simulink model "model_main_duty"  (R2024b)
settings: Solver=ode4  StartTime=0.0  StopTime=1000  FixedStep=dt  RelTol=1e-3
InitFcn:
  | model_init
undefined symbols (not defined in the file): dt, Iws, m_tot, norm_Ib, Omega1_init, Omega2_init, Omega3_init, Omega4_init, Omega_ref, qb0, rad2rpm, RCS_F, RCS_F_vec, RCS_Pos, RCS_pos, RCS_PWM_Freq, RCS_Sampling_time, RCS_THR_vec, REL_TS_POS_I_0, REL_TS_VEL_I_0, RW_As, RW_Max_Speed, RW_t_max, SC_Ib, SC_state0, SS_Total_Mass, TC_Kepler, TS_Ib, TS_qb0, TS_state0, TS_wb0, wb0
libraries: simulink_extras x17, simulink x16, sharedtransform x11, aerolibutil x10
(part 1 of 3)
settings Model: PacingRate=1.100000  Creator=yhj2019  LastModifiedBy=ASCL
settings DebuggingCC: UnderSpecifiedDimensionMsg=warning
settings RTWCC: GPUComputeCapability=3.5

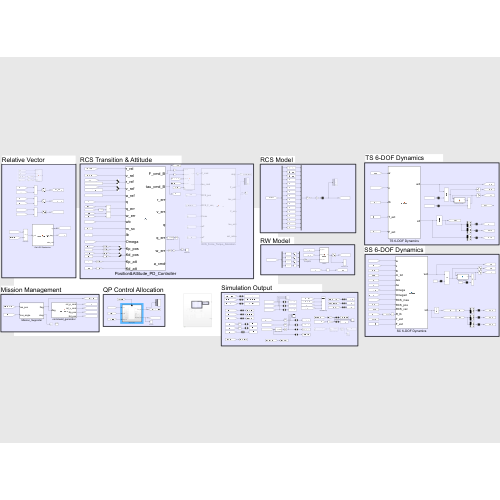
[thumbnail: Simulink's stored preview of the top-level diagram]
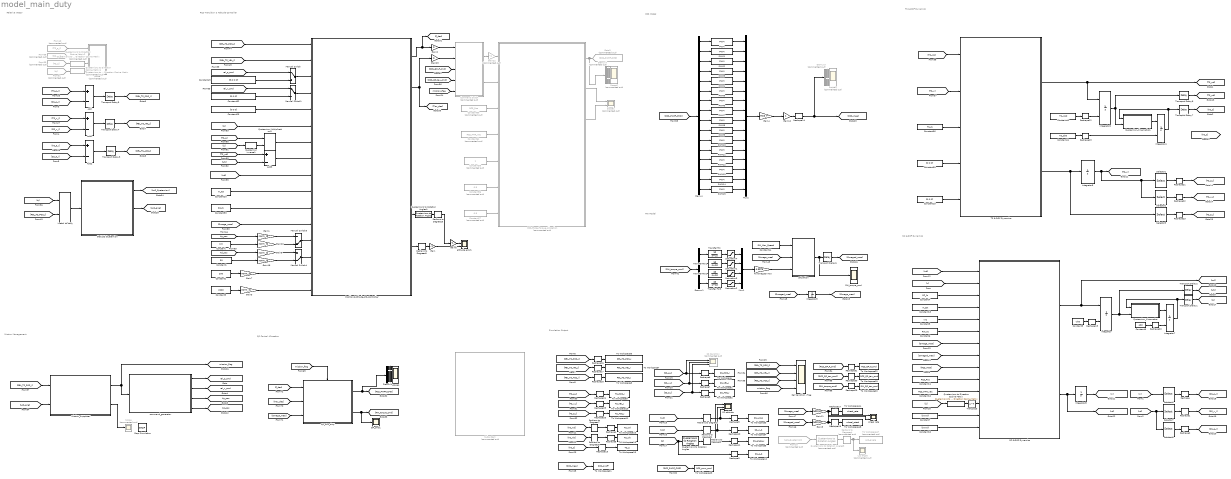
== system model_main_duty ==
  note: TS 6-DOF Dynamics
  note: RW Model
  note: RCS Model
  note: Simulation Output
  note: RCS Transition & Attitude Controller
  note: SS 6-DOF Dynamics
  note: Relative Vector
  note: Mission Management
  note: QP Control Allocation
  Add{,1..3} (4 alike) : Sum  Inputs=+-
  Command Switch : MATLAB Function  Commented=on  TreatAsAtomicUnit=on
  Constant : Constant  Value=0.3
  Constant1 : Constant  Value=30
  Constant{7,10,15,23,39,52} (6 alike) : Constant  Value=[0 0 0]'
  Constant11 : Constant  Value=RCS_Pos
  Constant12 : Constant  Value=RCS_THR_vec
  Constant13 : Constant  Value=m_tot
  Constant14 : Constant  Value=RW_Max_Speed
  Constant2 : Constant  Value=200
  Constant20 : Constant  Value=m_tot
  Constant3 : Constant  Value=2000
  Constant36 : Constant  Value=TS_Ib
  Constant4 : Constant  Value=SC_Ib
  Constant40 : Constant  Value=TS_wb0
  Constant41 : Constant  Value=TS_qb0
  Constant49 : Constant  Value=[5.0 0 0]'
  Constant5 : Constant  Value=Iws
  Constant53 : Constant  Value=SC_Ib
  Constant55 : Constant  Commented=on
  Constant56 : Constant  Commented=on  Value=0.5
  Constant57 : Constant  Commented=on  Value=0.5
  Constant6 : Constant  Value=RW_As
  Constant60 : Constant  Commented=on  Value=RCS_Pos
  Constant61 : Constant  Commented=on  Value=RCS_THR_vec
  Constant8 : Constant  Value=wb0
  Constant9 : Constant  Value=qb0
  Demux : Demux  Outputs=16
  Demux1 : Demux
  Demux2 : Demux  Commented=on  Outputs=16
  Demux3 : Demux  Commented=on  Outputs=16
  Demux4 : Demux  Outputs=16
  From10 : From  Commented=on  GotoTag=LoS_Quaternion
  From31 : From  Commented=on  GotoTag=q
  From39 : From  Commented=on  GotoTag=TS_q
  From40 : From  Commented=on  GotoTag=TS_p_I
  From68 : From  Commented=on  GotoTag=SS_p_I
  Gain : Gain  Gain=-1
  Gain{1,3,5,7,18,20} (6 alike) : Gain  Gain=norm_Ib
  Gain11 : Gain  Gain=rad2rpm
  Gain12 : Gain
  Gain2 : Gain  Gain=0
  Gain22 : Gain  Commented=on  Gain=-1
  Gain23 : Gain  Gain=0
  Gain4 : Gain  Gain=RCS_F
  Gain6 : Gain  Gain=-1
  Gain8 : Gain  Gain=rad2rpm
  Get LOS Quaternion : MATLAB Function  TreatAsAtomicUnit=on
  Goto3 : Goto  Commented=on  GotoTag=RCS_PWPF_CMD
  Inetial to body : aerolibutil/Quaternion Rotation
  Integrator : Integrator  InitialConditionSource=external  InitialCondition=wb0
  Integrator2 : Integrator  InitialConditionSource=external  InitialCondition=wb0
  Integrator3 : Integrator  InitialCondition=[Omega1_init Omega2_init Omega3_init Omega4_init]'
  Integrator4 : Integrator  InitialConditionSource=external
  Integrator5 : Integrator  InitialCondition=TS_state0'
  Integrator7 : Integrator  InitialConditionSource=external
  Integrator8 : Integrator  InitialCondition=SC_state0'
  Los angle : Scope  Commented=on
  Manual Switch : ManualSwitch
  Manual Switch1 : ManualSwitch
  Manual Switch3 : ManualSwitch  CurrentSetting=0
  Manual Switch4 : ManualSwitch  CurrentSetting=0
  Mission_Supporter : MATLAB Function  TreatAsAtomicUnit=on
  Mux1 : Mux
  Mux2 : Mux  Inputs=16
  PWM{,1..15} (16 alike) : simulink/Discontinuities/PWM  DisableCoverage=on  Period=RCS_PWM_Freq  InitialDelay=0  DisallowZeroDutyCycle=off  RunAtFixedTimeIntervals=on  SampleTime=RCS_Sampling_time
  Position&Attitude_PD_Controller : MATLAB Function  TreatAsAtomicUnit=on
  QP_RCS_duty : Subsystem  TreatAsAtomicUnit=on
  QP_cmd1 : Scope
  Quaternion Inverse1 : aerolibutil/Quaternion Inverse
  Quaternion Multiplication3 : aerolibutil/Quaternion Multiplication
  Quaternion_Kinematics : MATLAB Function  TreatAsAtomicUnit=on
  Quaternion_Kinematics1 : MATLAB Function  TreatAsAtomicUnit=on
  Quaternions to Direction Cosine Matrix : sharedtransform/Quaternions to  Direction Cosine Matrix  aMode=aMode
      settings: LibrarySourceBlock=|
      | aerolibtransform2/Quaternions to
      | Direction Cosine Matrix
  Quaternions to Direction Cosine Matrix1 : sharedtransform/Quaternions to  Direction Cosine Matrix  Commented=on  aMode=aMode
      settings: LibrarySourceBlock=|
      | aerolibtransform2/Quaternions to
      | Direction Cosine Matrix
  Quaternions to Direction Cosine Matrix2 : sharedtransform/Quaternions to  Direction Cosine Matrix  Commented=on  aMode=aMode
      settings: LibrarySourceBlock=|
      | aerolibtransform2/Quaternions to
      | Direction Cosine Matrix
  Quaternions to Rotation Angles : sharedtransform/Quaternions to Rotation Angles  rotationOrder=ZYX  aMode=aMode
  Quaternions to Rotation Angles1 : sharedtransform/Quaternions to Rotation Angles  rotationOrder=ZYX  aMode=aMode
  Quaternions to Rotation Angles3 : sharedtransform/Quaternions to Rotation Angles  Commented=on  rotationOrder=ZYX  aMode=aMode
  RCS_Force_Torque_Allocation : MATLAB Function  Commented=on  TreatAsAtomicUnit=on
  RW_torque_cmd : Scope
  Radians to Degrees{,1..3,7..9} (7 alike) : simulink_extras/Transformations/Radians to Degrees
  Radians to Degrees4 : simulink_extras/Transformations/Radians to Degrees  Commented=on
  Rel transition / flag : Scope  NumInputPorts=4
  Reshape{,1..2,12..14,19..23} (11 alike) : Reshape  OutputDimensionality=Column vector (2-D)
  Reshape{3..11,15..18,24..31} (21 alike) : Reshape  OutputDimensionality=Row vector (2-D)
  SC 6-DOF Dynamics : MATLAB Function  TreatAsAtomicUnit=on
  SS attitude : Scope  NumInputPorts=3
  SS transition : Scope  Commented=on  NumInputPorts=3
  Saturation{1..4} (4 alike) : Saturate  UpperLimit=RW_t_max  LowerLimit=-RW_t_max
  Scope : Scope  Commented=on
  Scope1 : Scope  Commented=on  NumInputPorts=2
  Scope2 : Scope  Commented=on  NumInputPorts=16
  Scope3 : Scope  Commented=on  NumInputPorts=16
  Scope4 : Scope  NumInputPorts=16
  Selector1 : Selector  InputPortWidth=6  IndexOptions=Index vector (dialog)  Indices=[1 2 3]  OutputSizes=1
  Selector2 : Selector  InputPortWidth=6  IndexOptions=Index vector (dialog)  Indices=[4 5 6]  OutputSizes=1
  Selector6 : Selector  InputPortWidth=6  IndexOptions=Index vector (dialog)  Indices=[1 2 3]  OutputSizes=1
  Selector7 : Selector  InputPortWidth=6  IndexOptions=Index vector (dialog)  Indices=[1 2 3]  OutputSizes=1
  Selector8 : Selector  InputPortWidth=6  IndexOptions=Index vector (dialog)  Indices=[4 5 6]  OutputSizes=1
  Selector9 : Selector  InputPortWidth=6  IndexOptions=Index vector (dialog)  Indices=[4 5 6]  OutputSizes=1
  Stop Simulation : Stop
  Subsystem : Subsystem  Commented=on
  TS 6-DOF Dynamics : MATLAB Function  TreatAsAtomicUnit=on
  To OmegaD max : Gain  Gain=4.3975
  To Workspace : ToWorkspace  VariableName=SS_POS_I  SampleTime=-1
      settings: Save2DSignal=2-D array (concatenate along first dimension)
  To Workspace1 : ToWorkspace  VariableName=SS_VEL_I  SampleTime=-1
      settings: Save2DSignal=2-D array (concatenate along first dimension)
  To Workspace10 : ToWorkspace  VariableName=TS_VEL_I  SampleTime=-1
      settings: Save2DSignal=2-D array (concatenate along first dimension)
  To Workspace11 : ToWorkspace  VariableName=TS_ACC_I  SampleTime=-1
      settings: Save2DSignal=2-D array (concatenate along first dimension)
  To Workspace12 : ToWorkspace  VariableName=SS_q_b  SampleTime=-1
      settings: Save2DSignal=2-D array (concatenate along first dimension)
  To Workspace13 : ToWorkspace  VariableName=TS_wb  SampleTime=-1
      settings: Save2DSignal=2-D array (concatenate along first dimension)
  To Workspace14 : ToWorkspace  VariableName=wheel_rate  SampleTime=-1
      settings: Save2DSignal=2-D array (concatenate along first dimension)
  To Workspace15 : ToWorkspace  VariableName=TS_q  SampleTime=-1
      settings: Save2DSignal=2-D array (concatenate along first dimension)
  To Workspace16 : ToWorkspace  VariableName=TS_wd  SampleTime=-1
      settings: Save2DSignal=2-D array (concatenate along first dimension)
  To Workspace17 : ToWorkspace  Commented=on  VariableName=LoS_angle  SampleTime=-1
      settings: Save2DSignal=2-D array (concatenate along first dimension)
  To Workspace18 : ToWorkspace  VariableName=wheel_rated  SampleTime=-1
      settings: Save2DSignal=2-D array (concatenate along first dimension)
  To Workspace19 : ToWorkspace  VariableName=RCS_QP_tau_cmd  SampleTime=-1
      settings: Save2DSignal=2-D array (concatenate along first dimension)
  To Workspace2 : ToWorkspace  VariableName=SS_ACC_I  SampleTime=-1
      settings: Save2DSignal=2-D array (concatenate along first dimension)
  To Workspace20 : ToWorkspace  VariableName=RW_QP_tau_cmd  SampleTime=-1
      settings: Save2DSignal=2-D array (concatenate along first dimension)
  To Workspace21 : ToWorkspace  VariableName=RCS_onoff  SaveFormat=Timeseries  SampleTime=-1
  To Workspace22 : ToWorkspace  VariableName=RCS_QP_F_cmd  SampleTime=-1
      settings: Save2DSignal=2-D array (concatenate along first dimension)
  To Workspace23 : ToWorkspace  VariableName=RCS_pwm_cmd  SaveFormat=Timeseries  SampleTime=-1
  To Workspace3 : ToWorkspace  VariableName=SS_wd_b  SampleTime=-1
      settings: Save2DSignal=2-D array (concatenate along first dimension)
  To Workspace4 : ToWorkspace  VariableName=SS_w_b  SampleTime=-1
      settings: Save2DSignal=2-D array (concatenate along first dimension)
  To Workspace5 : ToWorkspace  VariableName=SS_angle_I  SampleTime=-1
      settings: Save2DSignal=2-D array (concatenate along first dimension)
  To Workspace6 : ToWorkspace  VariableName=REL_TS_POS_I  SampleTime=-1
      settings: Save2DSignal=2-D array (concatenate along first dimension)
  To Workspace7 : ToWorkspace  VariableName=REL_TS_VEL_I  SampleTime=-1
      settings: Save2DSignal=2-D array (concatenate along first dimension)
  To Workspace8 : ToWorkspace  VariableName=REL_TS_ACC_I  SampleTime=-1
      settings: Save2DSignal=2-D array (concatenate along first dimension)
  To Workspace9 : ToWorkspace  VariableName=TS_POS_I  SampleTime=-1
      settings: Save2DSignal=2-D array (concatenate along first dimension)
  Transfer Fcn{,1..3} (4 alike) : TransferFcn  Numerator=[10]  Denominator=[1 10]
  Transport Delay1 : TransportDelay  DelayTime=dt  InitialOutput=qb0
  Transport Delay2 : TransportDelay  DelayTime=dt  InitialOutput=wb0
  Transport Delay3 : TransportDelay  DelayTime=dt  InitialOutput=[0 0 0]'
  Transport Delay4 : TransportDelay  DelayTime=dt  InitialOutput=REL_TS_VEL_I_0
  Transport Delay5 : TransportDelay  DelayTime=dt  InitialOutput=REL_TS_POS_I_0
  Transport Delay6 : TransportDelay  DelayTime=dt  InitialOutput=[0 0 0 0]'
  Transport Delay7 : TransportDelay  DelayTime=dt  InitialOutput=TS_qb0
  Transport Delay8 : TransportDelay  DelayTime=dt  InitialOutput=TS_wb0
  Transpose : Math  Operator=transpose
  attitude error1 : Scope  NumInputPorts=2
  command_generator : MATLAB Function  TreatAsAtomicUnit=on
  probe : MATLAB Function  Commented=on  TreatAsAtomicUnit=on
  saturation : MATLAB Function  TreatAsAtomicUnit=on
  wheel rate : Scope  NumInputPorts=2
  tag scope: Kd_pos=global, Kp_pos=global, mission_flag=global, rel_p_cmd=global, rel_v_cmd=global
  wires:
  Reshape6/1 -> To Workspace/1
  Reshape7/1 -> To Workspace1/1
  Reshape8/1 -> To Workspace2/1
  [TS_p_I] -> Add/1
  [SS_p_I] -> Add/2
  [SS_v_I] -> Add1/2
  [TS_v_I] -> Add1/1
  [SS_a_I] -> Add2/2
  [TS_a_I] -> Add2/1
  Add/1 -> Transport Delay5/1
  Add1/1 -> Transport Delay4/1
  Add2/1 -> Transport Delay3/1
  Constant4/1 -> SC 6-DOF Dynamics/3(Ib)
  Constant5/1 -> SC 6-DOF Dynamics/5(Iws)
  SC 6-DOF Dynamics/1(wd) -> [wd], Integrator/1
  [wb] -> SC 6-DOF Dynamics/1(w)
  Constant6/1 -> SC 6-DOF Dynamics/6(As)
  [Omega_mea] -> SC 6-DOF Dynamics/7(Omega)
  [Omegad_mea] -> SC 6-DOF Dynamics/8(Omegad)
  Quaternion_Kinematics/1(qd) -> Integrator7/1
  Constant8/1 -> Reshape19/1
  Constant9/1 -> Reshape20/1
  Quaternions to Rotation Angles/1 -> Radians to Degrees2/1
  [wd] -> Radians to Degrees/1
  [wb] -> Radians to Degrees1/1
  Radians to Degrees/1 -> SS attitude/3, Reshape9/1
  Radians to Degrees1/1 -> SS attitude/2, Reshape10/1
  Radians to Degrees2/1 -> SS attitude/1, Reshape11/1
  [q] -> Reshape3/1, Quaternions to Rotation Angles/1
  Constant10/1 -> SC 6-DOF Dynamics/14(F_ext)
  Constant13/1 -> SC 6-DOF Dynamics/4(m_tot)
  [q] -> Quaternions to Direction Cosine Matrix/1
  Quaternions to Direction Cosine Matrix/1 -> Transpose/1
  [SS_v_I] -> SS transition/2, Reshape7/1
  Transpose/1 -> SC 6-DOF Dynamics/12(R_Ib)
  Reshape9/1 -> To Workspace3/1
  Reshape10/1 -> To Workspace4/1
  Reshape11/1 -> To Workspace5/1
  SC 6-DOF Dynamics/2(xd) -> [xd], Integrator8/1
  Integrator8/1 -> [x]
  Selector8/1 -> Reshape2/1
  Selector6/1 -> Reshape/1
  [xd] -> Selector8/1, Selector7/1
  [x] -> Selector6/1
  Selector7/1 -> Reshape1/1
  [x] -> SC 6-DOF Dynamics/2(x)
  Constant11/1 -> SC 6-DOF Dynamics/10(RCS_pos)
  Constant12/1 -> SC 6-DOF Dynamics/11(RCS_vec)
  Demux/1 -> PWM/1
  Demux/2 -> PWM1/1
  Demux/3 -> PWM2/1
  Demux/4 -> PWM3/1
  Demux/8 -> PWM7/1
  Demux/5 -> PWM4/1
  Demux/6 -> PWM5/1
  Demux/7 -> PWM6/1
  Demux/14 -> PWM13/1
  Demux/13 -> PWM12/1
  Demux/15 -> PWM14/1
  Demux/12 -> PWM11/1
  Demux/16 -> PWM15/1
  Demux/9 -> PWM8/1
  Demux/10 -> PWM9/1
  Demux/11 -> PWM10/1
  PWM/1 -> Mux2/1
  Mux2/1 -> Gain4/1
  PWM1/1 -> Mux2/2
  PWM2/1 -> Mux2/3
  PWM3/1 -> Mux2/4
  PWM4/1 -> Mux2/5
  PWM5/1 -> Mux2/6
  PWM6/1 -> Mux2/7
  PWM7/1 -> Mux2/8
  PWM8/1 -> Mux2/9
  PWM9/1 -> Mux2/10
  PWM10/1 -> Mux2/11
  PWM11/1 -> Mux2/12
  PWM12/1 -> Mux2/13
  PWM13/1 -> Mux2/14
  PWM14/1 -> Mux2/15
  PWM15/1 -> Mux2/16
  [RCS_mea] -> SC 6-DOF Dynamics/9(RCS_mea)
  Gain4/1 -> Gain12/1
  Reshape/1 -> [SS_p_I]
  Reshape1/1 -> [SS_v_I]
  Reshape2/1 -> [SS_a_I]
  [REL_TS_POS_I] -> Reshape16/1
  [REL_TS_VEL_I] -> Reshape17/1
  [REL_TS_ACC_I] -> Reshape18/1
  Reshape16/1 -> To Workspace6/1
  Reshape17/1 -> To Workspace7/1
  Reshape18/1 -> To Workspace8/1
  [REL_TS_POS_I] -> Rel transition / flag/1
  [REL_TS_VEL_I] -> Rel transition / flag/2
  [REL_TS_ACC_I] -> Rel transition / flag/3
  Get LOS Quaternion/1(q) -> [LoS_Quaternion]  "LOS quaternion"
  [q] -> Inetial to body/1
  Inetial to body/1 -> Get LOS Quaternion/1(r_rel)
  [REL_TS_POS_I] -> Inetial to body/2
  Reshape19/1 -> Integrator/2
  Reshape20/1 -> Integrator7/2
  Gain12/1 -> Reshape14/1
  Demux1/1 -> Transfer Fcn/1
  Demux1/4 -> Transfer Fcn3/1
  Demux1/2 -> Transfer Fcn1/1
  Demux1/3 -> Transfer Fcn2/1
  Transfer Fcn/1 -> Saturation4/1
  Transfer Fcn1/1 -> Saturation1/1
  Transfer Fcn2/1 -> Saturation3/1
  Transfer Fcn3/1 -> Saturation2/1
  [Omegad_mea] -> Integrator3/1
  Integrator3/1 -> [Omega_mea]
  Integrator/1 -> Quaternion_Kinematics/2(w), Transport Delay2/1
  Integrator7/1 -> Quaternion_Kinematics/1(q), Transport Delay1/1
  [Omegad_mea] -> Gain8/1
  [Omega_mea] -> Gain11/1
  [RW_torque_cmd] -> Demux1/1
  saturation/1(res) -> RW_torque_cmd/1, Transport Delay6/1
  Saturation2/1 -> Mux1/4
  Saturation1/1 -> Mux1/2
  Saturation4/1 -> Mux1/1
  Saturation3/1 -> Mux1/3
  Mux1/1 -> To OmegaD max/1
  [Omega_mea] -> saturation/2(Omega_mea)
  Constant14/1 -> saturation/1(max_speed)
  [SS_p_I] -> SS transition/1, Reshape6/1
  [SS_a_I] -> SS transition/3, Reshape8/1
  Transport Delay1/1 -> [q]
  Transport Delay2/1 -> [wb]
  Transport Delay3/1 -> [REL_TS_ACC_I]
  Transport Delay4/1 -> [REL_TS_VEL_I]
  Transport Delay5/1 -> [REL_TS_POS_I]
  Transport Delay6/1 -> [Omegad_mea]
  Transport Delay7/1 -> [TS_q]
  Integrator4/1 -> Quaternion_Kinematics1/1(q), Transport Delay7/1
  Constant39/1 -> TS 6-DOF Dynamics/4(T_ext)
  Integrator2/1 -> Quaternion_Kinematics1/2(w), Transport Delay8/1
  Constant41/1 -> Reshape13/1
  Transport Delay8/1 -> [TS_wb]
  Integrator5/1 -> Selector2/1, Selector1/1, [TS_x]
  Reshape13/1 -> Integrator4/2
  TS 6-DOF Dynamics/2(xd) -> Selector9/1, Integrator5/1
  [TS_x] -> TS 6-DOF Dynamics/2(x)
  Quaternion_Kinematics1/1(qd) -> Integrator4/1
  Constant15/1 -> TS 6-DOF Dynamics/5(F_ext)
  TS 6-DOF Dynamics/1(wd) -> [TS_wd], Integrator2/1
  Constant40/1 -> Reshape12/1
  [TS_wb] -> TS 6-DOF Dynamics/1(w)
  Constant36/1 -> TS 6-DOF Dynamics/3(Ib)
  Reshape12/1 -> Integrator2/2
  Reshape21/1 -> [TS_p_I]
  Selector1/1 -> Reshape21/1
  Reshape22/1 -> [TS_v_I]
  Reshape23/1 -> [TS_a_I]
  Selector9/1 -> Reshape23/1
  Selector2/1 -> Reshape22/1
  [TS_v_I] -> Reshape25/1
  [TS_a_I] -> Reshape26/1
  Reshape25/1 -> To Workspace10/1
  Reshape24/1 -> To Workspace9/1
  Reshape26/1 -> To Workspace11/1
  [TS_p_I] -> Reshape24/1
  Reshape3/1 -> To Workspace12/1
  Radians to Degrees4/1 -> To Workspace17/1, Los angle/1
  Quaternions to Rotation Angles3/1 -> Radians to Degrees4/1
  [TS_wd] -> Radians to Degrees7/1
  Reshape15/1 -> To Workspace15/1
  Reshape4/1 -> To Workspace16/1
  Reshape5/1 -> To Workspace13/1
  [TS_wb] -> Radians to Degrees8/1
  Gain7/1 -> Position&Attitude_PD_Controller/15(Kp_att)
  Position&Attitude_PD_Controller/2(tau_cmd_B) -> [Tau_des], Gain23/1
  Constant20/1 -> Position&Attitude_PD_Controller/10(m_sc)
  [REL_TS_POS_I] -> Position&Attitude_PD_Controller/1(r_rel)
  Constant61/1 -> RCS_Force_Torque_Allocation/4(RCS_F_vec)
  Constant56/1 -> RCS_Force_Torque_Allocation/6(wF)
  Constant1/1 -> Gain18/1
  [q] -> Position&Attitude_PD_Controller/6("q ")
  [REL_TS_VEL_I] -> Position&Attitude_PD_Controller/2(v_rel)
  Position&Attitude_PD_Controller/1(F_cmd_B) -> [F_des], Gain2/1
  Gain3/1 -> Position&Attitude_PD_Controller/16(Kd_att)
  Constant23/1 -> Position&Attitude_PD_Controller/5(a_ref)
  RCS_Force_Torque_Allocation/1(duty) -> Demux2/1, Goto3/1
  Constant55/1 -> RCS_Force_Torque_Allocation/5(Fmax)
  Constant2/1 -> Gain7/1
  Constant/1 -> Gain20/1
  Constant57/1 -> RCS_Force_Torque_Allocation/7(wT)
  Constant60/1 -> RCS_Force_Torque_Allocation/3(RCS_pos)
  Gain22/1 -> RCS_Force_Torque_Allocation/1(F_cmd)
  [RCS_PWPF_CMD] -> Demux/1
  Constant53/1 -> Position&Attitude_PD_Controller/11(Ib)
  [wb] -> Position&Attitude_PD_Controller/9(wb)
  Constant3/1 -> Gain3/1
  Constant7/1 -> SC 6-DOF Dynamics/13(T_ext)
  [REL_TS_POS_I] -> Mission_Supporter/1(res_pos)
  Manual Switch1/1 -> Position&Attitude_PD_Controller/4(v_ref)
  Manual Switch/1 -> Position&Attitude_PD_Controller/3(r_ref)
  Constant52/1 -> Manual Switch1/2
  Constant49/1 -> Manual Switch/2
  Mission_Supporter/1(flag) -> command_generator/1(flag), [mission_flag]
  Manual Switch4/1 -> Position&Attitude_PD_Controller/14(Kd_pos)
  Gain18/1 -> Manual Switch4/2
  Gain20/1 -> Manual Switch3/2
  command_generator/4(Kd_pos) -> [Kd_pos]
  command_generator/3(Kp_pos) -> [Kp_pos]
  command_generator/2(rel_v_cmd) -> [rel_v_cmd]
  command_generator/1(rel_p_cmd) -> [rel_p_cmd]
  [rel_v_cmd] -> Manual Switch1/1
  [rel_p_cmd] -> Manual Switch/1
  [mission_flag] -> Rel transition / flag/4
  Mission_Supporter/2(stop) -> Scope/1
  [Kp_pos] -> Gain1/1
  [Kd_pos] -> Gain5/1
  Gain5/1 -> Manual Switch4/1
  Gain1/1 -> Manual Switch3/1
  From10/1 -> Quaternions to Rotation Angles3/1
  Manual Switch3/1 -> Position&Attitude_PD_Controller/13(Kp_pos)
  Command Switch/2(tau_cmd) -> RCS_Force_Torque_Allocation/2(tau_cmd)
  Gain11/1 -> wheel rate/1, Reshape27/1
  Reshape27/1 -> To Workspace14/1
  Gain8/1 -> wheel rate/2, Reshape28/1
  Reshape28/1 -> To Workspace18/1
  [LoS_ang] -> Mission_Supporter/2(Los_angle)
  Get LOS Quaternion/2(ang_deg) -> [LoS_ang]
  To OmegaD max/1 -> saturation/3(torque_cmd)
  Radians to Degrees7/1 -> Reshape4/1
  Radians to Degrees8/1 -> Reshape5/1
  [TS_q] -> Reshape15/1
  Command Switch/1(F_cmd) -> Gain22/1
  Gain23/1 -> Command Switch/2(tau_PD_cmd)
  Gain2/1 -> Command Switch/1(F_PD_cmd)
  [RCS_QP_tau_cmd] -> Command Switch/4(tau_QP_cmd)
  [RCS_QP_F_cmd] -> Command Switch/3(F_QP_cmd)
  [mission_flag] -> Command Switch/5(flag)
  [TS_wb] -> Add3/1
  [TS_q] -> Quaternion Multiplication3/1
  Quaternion Multiplication3/1 -> Position&Attitude_PD_Controller/7("q_err ")
  [wb] -> Add3/2
  Quaternion Inverse1/1 -> Quaternion Multiplication3/2
  [q] -> Quaternion Inverse1/1
  Add3/1 -> Position&Attitude_PD_Controller/8("w_err ")
  [Omega_mea] -> Position&Attitude_PD_Controller/12(Omega)
  Quaternions to Rotation Angles1/1 -> Radians to Degrees3/1
  [RCS_QP_F_cmd] -> Reshape31/1
  [RCS_QP_tau_cmd] -> Reshape30/1
  [RW_torque_cmd] -> Reshape29/1
  Reshape29/1 -> To Workspace20/1
  Reshape30/1 -> To Workspace19/1
  Reshape31/1 -> To Workspace22/1
  Position&Attitude_PD_Controller/7(w_err) -> Radians to Degrees9/1
  Position&Attitude_PD_Controller/6(q_err) -> Quaternions to Rotation Angles1/1
  Radians to Degrees3/1 -> Gain6/1
  Radians to Degrees9/1 -> Gain/1
  [RCS_mea] -> To Workspace21/1
  [RCS_PWPF_CMD] -> To Workspace23/1
  From31/1 -> Quaternions to Direction Cosine Matrix1/1
  From39/1 -> Quaternions to Direction Cosine Matrix2/1
  Quaternions to Direction Cosine Matrix1/1 -> probe/4(dcm_S)
  Quaternions to Direction Cosine Matrix2/1 -> probe/3(dcm_T)
  From40/1 -> probe/1(TS_p_I)
  From68/1 -> probe/2(SS_p_I)
  RCS_Force_Torque_Allocation/2(F_est) -> Scope1/1  "F_est"
  RCS_Force_Torque_Allocation/3(tau_est) -> Scope1/2  "Tau_est"
  [mission_flag] -> QP_RCS_duty/Enable
  [Omega_mea] -> QP_RCS_duty/3(Omega_mea)
  [F_des] -> QP_RCS_duty/1(F_des)
  QP_RCS_duty/2(RW_torque_cmd) -> [RW_torque_cmd], QP_cmd1/1
  [Tau_des] -> QP_RCS_duty/2(Tau_des)
  Demux2/1 -> Scope2/1
  Demux2/2 -> Scope2/2
  Demux2/3 -> Scope2/3
  Demux2/4 -> Scope2/4
  Demux2/5 -> Scope2/5
  Demux2/6 -> Scope2/6
  Demux2/7 -> Scope2/7
  Demux2/8 -> Scope2/8
  Demux2/9 -> Scope2/9
  Demux2/10 -> Scope2/10
  Demux2/11 -> Scope2/11
  Demux2/12 -> Scope2/12
  Demux2/13 -> Scope2/13
  Demux2/14 -> Scope2/14
  Demux2/15 -> Scope2/15
  Demux2/16 -> Scope2/16
  Gain/1 -> attitude error1/2
  Gain6/1 -> attitude error1/1
  Reshape14/1 -> Demux3/1, [RCS_mea]
  Demux3/14 -> Scope3/14
  Demux3/13 -> Scope3/13
  Demux3/16 -> Scope3/16
  Demux3/15 -> Scope3/15
  Demux3/11 -> Scope3/11
  Demux3/9 -> Scope3/9
  Demux3/10 -> Scope3/10
  Demux3/12 -> Scope3/12
  Demux3/7 -> Scope3/7
  Demux3/5 -> Scope3/5
  Demux3/4 -> Scope3/4
  Demux3/6 -> Scope3/6
  Demux3/3 -> Scope3/3
  Demux3/2 -> Scope3/2
  Demux3/1 -> Scope3/1
  Demux3/8 -> Scope3/8
  Demux4/13 -> Scope4/13
  Demux4/5 -> Scope4/5
  Demux4/2 -> Scope4/2
  Demux4/6 -> Scope4/6
  Demux4/3 -> Scope4/3
  Demux4/10 -> Scope4/10
  Demux4/9 -> Scope4/9
  Demux4/15 -> Scope4/15
  Demux4/12 -> Scope4/12
  Demux4/16 -> Scope4/16
  QP_RCS_duty/1(RCS_duty) -> Demux4/1, [RCS_PWPF_CMD]
  Demux4/11 -> Scope4/11
  Demux4/14 -> Scope4/14
  Demux4/1 -> Scope4/1
  Demux4/8 -> Scope4/8
  Demux4/7 -> Scope4/7
  Demux4/4 -> Scope4/4

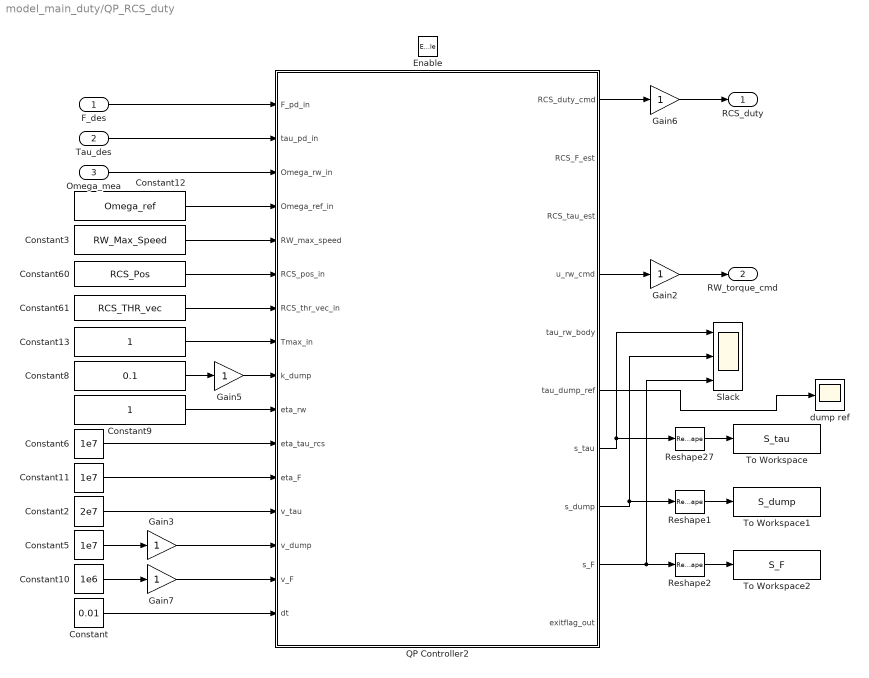
== system model_main_duty/QP_RCS_duty ==
  F_des : Inport
  Tau_des : Inport  Port=2
  Omega_mea : Inport  Port=3
  Enable : EnablePort
  Constant : Constant  Value=0.01
  Constant10 : Constant  Value=1e6
  Constant11 : Constant  Value=1e7
  Constant12 : Constant  Value=Omega_ref
  Constant13 : Constant
  Constant2 : Constant  Value=2e7
  Constant3 : Constant  Value=RW_Max_Speed
  Constant5 : Constant  Value=1e7
  Constant6 : Constant  Value=1e7
  Constant60 : Constant  Value=RCS_Pos
  Constant61 : Constant  Value=RCS_THR_vec
  Constant8 : Constant  Value=0.1
  Constant9 : Constant
  Gain{2..3,5..7} (5 alike) : Gain
  QP Controller2 : MATLAB Function  TreatAsAtomicUnit=on
  Reshape1 : Reshape  OutputDimensionality=Row vector (2-D)
  Reshape2 : Reshape  OutputDimensionality=Row vector (2-D)
  Reshape27 : Reshape  OutputDimensionality=Row vector (2-D)
  Slack : Scope  NumInputPorts=3
  To Workspace : ToWorkspace  VariableName=S_tau  SampleTime=-1
  To Workspace1 : ToWorkspace  VariableName=S_dump  SampleTime=-1
  To Workspace2 : ToWorkspace  VariableName=S_F  SampleTime=-1
  dump ref : Scope
  RCS_duty : Outport
  RW_torque_cmd : Outport  Port=2
  wires:
  QP Controller2/4(u_rw_cmd) -> Gain2/1
  Tau_des/1 -> QP Controller2/2(tau_pd_in)
  Omega_mea/1 -> QP Controller2/3(Omega_rw_in)
  Constant3/1 -> QP Controller2/5(RW_max_speed)
  Constant2/1 -> QP Controller2/13(v_tau)
  Constant6/1 -> QP Controller2/11(eta_tau_rcs)
  Constant5/1 -> Gain3/1
  Constant/1 -> QP Controller2/16(dt)
  Gain2/1 -> RW_torque_cmd/1
  Gain3/1 -> QP Controller2/14(v_dump)
  Constant12/1 -> QP Controller2/4(Omega_ref_in)
  Constant8/1 -> Gain5/1
  Constant9/1 -> QP Controller2/10(eta_rw)
  Gain5/1 -> QP Controller2/9(k_dump)
  F_des/1 -> QP Controller2/1(F_pd_in)
  QP Controller2/1(RCS_duty_cmd) -> Gain6/1
  Gain6/1 -> RCS_duty/1
  Constant10/1 -> Gain7/1
  Gain7/1 -> QP Controller2/15(v_F)
  Constant11/1 -> QP Controller2/12(eta_F)
  QP Controller2/7(s_tau) -> Slack/1, Reshape27/1
  QP Controller2/8(s_dump) -> Reshape1/1, Slack/2
  QP Controller2/9(s_F) -> Reshape2/1, Slack/3
  Reshape27/1 -> To Workspace/1
  Reshape1/1 -> To Workspace1/1
  Reshape2/1 -> To Workspace2/1
  Constant61/1 -> QP Controller2/7(RCS_thr_vec_in)
  QP Controller2/6(tau_dump_ref) -> dump ref/1
  Constant13/1 -> QP Controller2/8(Tmax_in)
  Constant60/1 -> QP Controller2/6(RCS_pos_in)

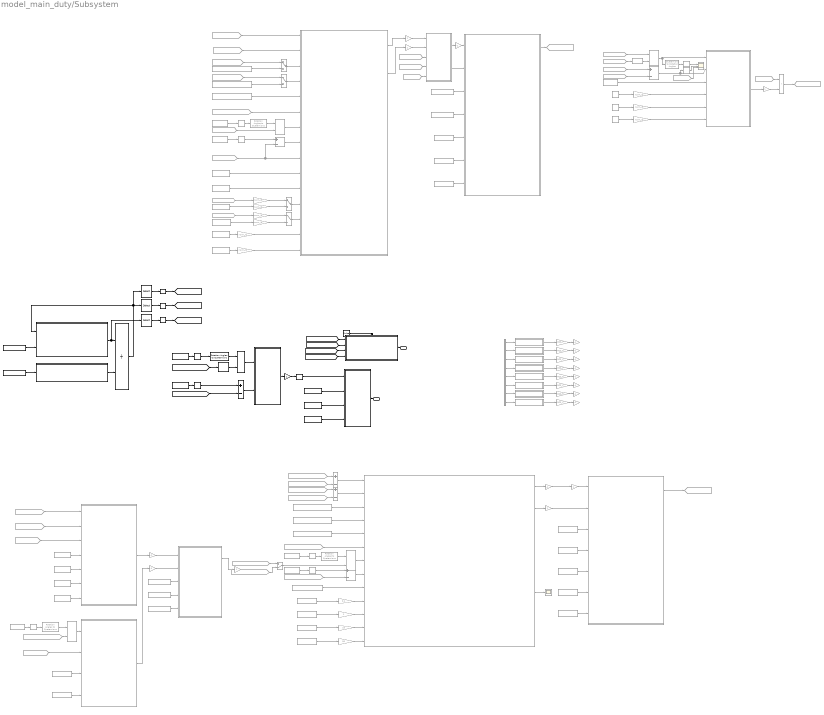
== system model_main_duty/Subsystem ==
  note: pwpfm
  note: RW Attitude Controller
  note: RCS Transition & Attitude Controller
  Add{4,6,10,12,15} (5 alike) : Sum  Commented=on  Inputs=+-
  Add3 : Sum  Inputs=+-
  Attitude_PD_control : MATLAB Function  TreatAsAtomicUnit=on
  Attitude_PD_control1 : MATLAB Function  Commented=on  TreatAsAtomicUnit=on
  Attitude_PD_control2 : MATLAB Function  Commented=on  TreatAsAtomicUnit=on
  Command Switch1 : MATLAB Function  Commented=on  TreatAsAtomicUnit=on
  Constant1 : Constant  Value=TC_Kepler
  Constant10 : Constant  Commented=on  Value=18
  Constant11 : Constant  Commented=on  Value=400
  Constant12 : Constant  Commented=on  Value=15000
  Constant13 : Constant  Commented=on  Value=0.01
  Constant14 : Constant  Commented=on  Value=200
  Constant15 : Constant  Commented=on  Value=m_tot
  Constant16 : Constant  Value=[45 0 0]
  Constant17 : Constant  Value=[0 0 0]
  Constant18 : Constant  Value=RCS_F
  Constant19 : Constant  Value=RCS_THR_vec
  Constant{2,40..41,50..51} (5 alike) : Constant  Commented=on  Value=[0 0 0]
  Constant20 : Constant  Value=RCS_Pos
  Constant21 : Constant  Commented=on  Value=SC_Ib
  Constant{6,22..25,32,43} (7 alike) : Constant  Commented=on  Value=[0 0 0]'
  Constant26 : Constant  Commented=on  Value=[2 0 0]'
  Constant27 : Constant  Commented=on  Value=RCS_Pos
  Constant28 : Constant  Commented=on  Value=RCS_THR_vec
  Constant29 : Constant  Commented=on  Value=RCS_F
  Constant3 : Constant  Value=[0 0 0]'
  Constant30 : Constant  Commented=on  Value=2000
  Constant31 : Constant  Commented=on  Value=[5.0 0 0]'
  Constant33 : Constant  Commented=on  Value=SC_Ib
  Constant34 : Constant  Commented=on
  Constant{35,39,47..48} (4 alike) : Constant  Commented=on  Value=0.5
  Constant36 : Constant  Commented=on  Value=RW_As
  Constant{4,8,37..38} (4 alike) : Constant  Commented=on  Value=diag([1 1 1])
  Constant42 : Constant  Commented=on  Value=[1.5 0 0]'
  Constant44 : Constant  Commented=on  Value=RCS_pos
  Constant45 : Constant  Commented=on  Value=RCS_F_vec
  Constant46 : Constant  Commented=on
  Constant49 : Constant  Commented=on  Value=RCS_Pos
  Constant5 : Constant  Commented=on  Value=SS_Total_Mass
  Constant52 : Constant  Commented=on  Value=RCS_THR_vec
  Constant7 : Constant  Commented=on  Value=m_tot
  Constant9 : Constant  Commented=on  Value=0.3
  Degrees to Radians1 : simulink_extras/Transformations/Degrees to Radians
  Degrees to Radians{2,4..7} (5 alike) : simulink_extras/Transformations/Degrees to Radians  Commented=on
  Degrees to Radians3 : simulink_extras/Transformations/Degrees to Radians
  Demux2 : Demux  Commented=on  Outputs=8
  From1 : From  Commented=on  GotoTag=LoS_Quaternion
  From12 : From  Commented=on  GotoTag=wb
  From2 : From  Commented=on  GotoTag=SS_LVLH_Attitude_Quaternion
  From3 : From  Commented=on  GotoTag=SS_Body_Position_ECI
  From30 : From  Commented=on  GotoTag=wb
  From31 : From  Commented=on  GotoTag=q
  From32 : From  Commented=on  GotoTag=REL_TS_POS_I
  From33 : From  Commented=on  GotoTag=REL_TS_VEL_I
  From39 : From  Commented=on  GotoTag=TS_Position
  From4 : From  Commented=on  GotoTag=mission_flag  TagVisibility=global
  From40 : From  Commented=on  GotoTag=wb
  From5 : From  Commented=on  GotoTag=TS_wb
  From56 : From  Commented=on  GotoTag=SS_ECI_Attitude_Quaternion
  From6 : From  Commented=on  GotoTag=TS_q
  From61 : From  Commented=on  GotoTag=SS_Body_Angular_Rate
  From62 : From  Commented=on  GotoTag=LoS_Quaternion
  From68 : From  Commented=on  GotoTag=mission_flag  TagVisibility=global
  From69 : From  Commented=on  GotoTag=SS_Body_Velocity_ECI
  From7 : From  Commented=on  GotoTag=q
  From70 : From  Commented=on  GotoTag=REL_TS_VEL_I
  From71 : From  Commented=on  GotoTag=q
  From72 : From  Commented=on  GotoTag=TS_Velocity
  From73 : From  Commented=on  GotoTag=RCS_QP_tau_cmd
  From74 : From  Commented=on  GotoTag=rel_p_cmd  TagVisibility=global
  From75 : From  Commented=on  GotoTag=LoS_Quaternion
  From76 : From  Commented=on  GotoTag=RCS_QP_F_cmd
  From77 : From  Commented=on  GotoTag=rel_v_cmd  TagVisibility=global
  From78 : From  Commented=on  GotoTag=Kp_pos  TagVisibility=global
  From79 : From  Commented=on  GotoTag=Kd_pos  TagVisibility=global
  From8 : From  Commented=on  GotoTag=mission_flag  TagVisibility=global
  From9 : From  Commented=on  GotoTag=REL_TS_POS_I
  Gain{,24..27,36..38} (8 alike) : Gain  Commented=on  Gain=RCS_F
  Gain1 : Gain  Commented=on  Gain=0
  Gain{2,8..10,12,16,19} (7 alike) : Gain  Commented=on
  Gain{3..4,7,11,18,20,22..23,39} (9 alike) : Gain  Commented=on  Gain=norm_Ib
  Gain{6,13,21,28..35} (11 alike) : Gain  Commented=on  Gain=-1
  Gain14 : Gain  Commented=on  Gain=50
  Gain15 : Gain  Commented=on  Gain=10
  Gain17 : Gain  Commented=on  Gain=0.1
  Gain5 : Gain
  Get LOS Quaternion7 : MATLAB Function  Commented=on  TreatAsAtomicUnit=on
  Goto32 : Goto  Commented=on  GotoTag=Tau_des
  Goto33 : Goto  Commented=on  GotoTag=RCS_PWPF_CMD
  Goto42 : Goto  Commented=on  GotoTag=RCS_PWPF_CMD
  Integrator1 : Integrator  InitialConditionSource=external  InitialCondition=[-7000 0 0 0 -9.175045 0 5233.5]'
  MATLAB Function1 : MATLAB Function  TreatAsAtomicUnit=on
  Manual Switch{1,5..7} (4 alike) : ManualSwitch  Commented=on
  Manual Switch2 : ManualSwitch  Commented=on  CurrentSetting=0
  Product1 : Product  Commented=on
  Pulse Generator : DiscretePulseGenerator  PulseType=Time based  Period=0.2  PulseWidth=50
  Quaternion Inverse : aerolibutil/Quaternion Inverse
  Quaternion Inverse1 : aerolibutil/Quaternion Inverse  Commented=on
  Quaternion Multiplication : aerolibutil/Quaternion Multiplication
  Quaternion Multiplication{1..4} (4 alike) : aerolibutil/Quaternion Multiplication  Commented=on
  Quaternions to Rotation Angles2 : sharedtransform/Quaternions to Rotation Angles  Commented=on  rotationOrder=ZYX  aMode=aMode
  RCS_Controller : Subsystem
  RCS_Force_Torque_Allocation1 : MATLAB Function  Commented=on  TreatAsAtomicUnit=on
  RCS_Position&Attitude_Controller1 : MATLAB Function  Commented=on  TreatAsAtomicUnit=on
  RCS_Relative_Position_Control_Allocation1 : MATLAB Function  Commented=on  TreatAsAtomicUnit=on
  Radians to Degrees5 : simulink_extras/Transformations/Radians to Degrees  Commented=on
  Radians to Degrees6 : simulink_extras/Transformations/Radians to Degrees  Commented=on
  Reshape{3..5,15} (4 alike) : Reshape  OutputDimensionality=Column vector (2-D)
  Rotation Angles to Quaternions1 : sharedtransform/Rotation Angles to Quaternions  rotationOrder=ZYX  aMode=aMode
  Rotation Angles to Quaternions2 : sharedtransform/Rotation Angles to Quaternions  Commented=on  rotationOrder=ZYX  aMode=aMode
  Rotation Angles to Quaternions3 : sharedtransform/Rotation Angles to Quaternions  Commented=on  rotationOrder=ZYX  aMode=aMode
  Rotation Angles to Quaternions4 : sharedtransform/Rotation Angles to Quaternions  Commented=on  rotationOrder=ZYX  aMode=aMode
  SS Attitude Control wrt ECI : MATLAB Function  Commented=on  TreatAsAtomicUnit=on
  Scope7 : Scope  Commented=on
  Selector3 : Selector  InputPortWidth=6  IndexOptions=Index vector (dialog)  Indices=[1 2 3]  OutputSizes=1
  Selector4 : Selector  InputPortWidth=6  IndexOptions=Index vector (dialog)  Indices=[4 5 6]  OutputSizes=1
  Selector5 : Selector  InputPortWidth=6  IndexOptions=Index vector (dialog)  Indices=[4 5 6]  OutputSizes=1
  Subsystem1 : Subsystem  Commented=on
  Subsystem2 : Subsystem  Commented=on
  Subsystem3 : Subsystem  Commented=on
  Subsystem4 : Subsystem  Commented=on
  Subsystem5 : Subsystem  Commented=on
  Subsystem6 : Subsystem  Commented=on
  Subsystem7 : Subsystem  Commented=on
  Subsystem8 : Subsystem  Commented=on
  TC Kepler Propagate : MATLAB Function  TreatAsAtomicUnit=on
  THR_Allocation : MATLAB Function  TreatAsAtomicUnit=on
  Thruster Allocation : MATLAB Function  Commented=on  TreatAsAtomicUnit=on
  attitude error : Scope  Commented=on  NumInputPorts=3
  u : Outport
  pwm : Outport  Port=2
  wires:
  Reshape15/1 -> THR_Allocation/1(tau_cmd)
  Selector4/1 -> Reshape4/1
  TC Kepler Propagate/1(dfdt) -> Selector5/1, Integrator1/1
  Pulse Generator/1 -> RCS_Controller/Trigger
  [SC_quat_LVLH] -> RCS_Controller/3(SC_quat_LVLH)
  Constant16/1 -> Degrees to Radians1/1
  Quaternion Multiplication/1 -> Attitude_PD_control/1(q_err)
  [q] -> Quaternion Inverse/1
  Selector5/1 -> Reshape5/1
  Gain5/1 -> Reshape15/1
  [SC_rate_LVLH] -> RCS_Controller/4(SC_rate_LVLH)
  Constant1/1 -> MATLAB Function1/1(kepel)
  Attitude_PD_control/1(u_torq) -> Gain5/1
  [SC_Position_mea] -> RCS_Controller/1(SC_Position_mea)
  Constant17/1 -> Degrees to Radians3/1
  Integrator1/1 -> Selector3/1, TC Kepler Propagate/1(initial_condition), Selector4/1
  Constant19/1 -> THR_Allocation/3(f)
  MATLAB Function1/1(statvec) -> Integrator1/2
  Constant20/1 -> THR_Allocation/4(r_thr)
  Reshape5/1 -> [TS_a_I]
  Constant3/1 -> TC Kepler Propagate/2(F_eci)
  [SC_Velocity_mea] -> RCS_Controller/2(SC_Velocity_mea)
  Degrees to Radians1/1 -> Rotation Angles to Quaternions1/1
  Rotation Angles to Quaternions1/1 -> Quaternion Multiplication/1
  [wb] -> Add3/2
  Constant18/1 -> THR_Allocation/2(F_on)
  Selector3/1 -> Reshape3/1
  Reshape4/1 -> [TS_v_I]
  Add3/1 -> Attitude_PD_control/2(w_err)
  Reshape3/1 -> [TS_p_I]
  Degrees to Radians3/1 -> Add3/1
  Quaternion Inverse/1 -> Quaternion Multiplication/2
  RCS_Controller/1(u) -> u/1
  THR_Allocation/1(pwm) -> pwm/1
  Get LOS Quaternion7/1(F_cmd_B) -> Gain13/1
  Add12/1 -> Get LOS Quaternion7/8("w_err ")
  Constant7/1 -> Attitude_PD_control1/7(m)
  Degrees to Radians6/1 -> Rotation Angles to Quaternions3/1
  Constant8/1 -> Gain15/1
  Quaternion Multiplication2/1 -> Attitude_PD_control2/1(q_err)
  From2/1 -> Manual Switch2/1
  Quaternion Multiplication3/1 -> Get LOS Quaternion7/7(q_err)
  Gain13/1 -> Gain2/1
  Gain14/1 -> Get LOS Quaternion7/13(Kd_att)
  Rotation Angles to Quaternions3/1 -> Quaternion Multiplication3/1
  Manual Switch2/1 -> Quaternion Multiplication3/2
  Gain2/1 -> RCS_Relative_Position_Control_Allocation1/1(F_cmd)
  Add6/1 -> Get LOS Quaternion7/1(r_rel)
  From31/1 -> Attitude_PD_control1/3(q_IB)
  Constant22/1 -> Attitude_PD_control2/3(omega_d_B)
  From39/1 -> Add6/1
  From3/1 -> Add6/2
  Constant27/1 -> Thruster Allocation/3(r)
  Constant28/1 -> Thruster Allocation/4(d)
  Constant2/1 -> Degrees to Radians2/1
  Attitude_PD_control2/1(tau_B_cmd) -> Gain1/1
  Constant46/1 -> RCS_Relative_Position_Control_Allocation1/5(Tmax)
  RCS_Relative_Position_Control_Allocation1/1(duty) -> Goto42/1
  Constant6/1 -> Get LOS Quaternion7/5(a_ref)
  Get LOS Quaternion7/2(tau_cmd_B) -> Gain19/1
  Constant51/1 -> Degrees to Radians7/1
  From32/1 -> Attitude_PD_control1/1(r_I)
  Constant37/1 -> Gain17/1
  Constant47/1 -> RCS_Relative_Position_Control_Allocation1/6(wF)
  From30/1 -> Attitude_PD_control2/2(omega_B)
  Constant43/1 -> Get LOS Quaternion7/4(v_ref)
  Constant29/1 -> Thruster Allocation/5(F_max)
  Constant26/1 -> Attitude_PD_control1/4(r_d)
  Rotation Angles to Quaternions2/1 -> Quaternion Multiplication2/1
  Constant50/1 -> Degrees to Radians6/1
  From1/1 -> Quaternion Multiplication2/2
  From62/1 -> Manual Switch2/2
  Constant21/1 -> Attitude_PD_control2/4(J)
  Constant44/1 -> RCS_Relative_Position_Control_Allocation1/3(RCS_pos)
  From72/1 -> Add15/1
  Gain16/1 -> Get LOS Quaternion7/11(Kd_pos)
  Degrees to Radians2/1 -> Rotation Angles to Quaternions2/1
  Gain6/1 -> Thruster Allocation/1(F_B_cmd)
  Get LOS Quaternion7/6(q_err_vec) -> Scope7/1
  From56/1 -> Get LOS Quaternion7/6("q ")
  From69/1 -> Add15/2
  Attitude_PD_control1/1(F_B_cmd) -> Gain6/1
  Thruster Allocation/1(u_pwm) -> Gain9/1
  Gain1/1 -> Thruster Allocation/2(tau_B_cmd)
  Degrees to Radians7/1 -> Add12/1
  Gain19/1 -> RCS_Relative_Position_Control_Allocation1/2(tau_cmd)
  From61/1 -> Add12/2
  Constant5/1 -> Get LOS Quaternion7/9(m_sc)
  Constant25/1 -> Attitude_PD_control1/5(v_d)
  Constant24/1 -> Attitude_PD_control1/6(a_d)
  From33/1 -> Attitude_PD_control1/2(v_I)
  Constant38/1 -> Gain16/1
  Constant48/1 -> RCS_Relative_Position_Control_Allocation1/7(wT)
  Constant4/1 -> Gain14/1
  Constant45/1 -> RCS_Relative_Position_Control_Allocation1/4(RCS_F_vec)
  Gain15/1 -> Get LOS Quaternion7/12(Kp_att)
  Gain17/1 -> Get LOS Quaternion7/10(Kp_pos)
  Constant42/1 -> Get LOS Quaternion7/3(r_ref)
  Add15/1 -> Get LOS Quaternion7/2(v_rel)
  Demux2/4 -> Subsystem4/1(In1)
  Demux2/5 -> Subsystem5/1(In1)
  Subsystem2/1(F_gated) -> Gain36/1
  Gain26/1 -> Gain34/1
  Gain38/1 -> Gain31/1
  Demux2/7 -> Subsystem7/1(In1)
  Gain27/1 -> Gain35/1
  Subsystem6/1(F_gated) -> Gain25/1
  Demux2/3 -> Subsystem3/1(In1)
  Subsystem3/1(F_gated) -> Gain37/1
  Demux2/6 -> Subsystem6/1(In1)
  Subsystem7/1(F_gated) -> Gain26/1
  Gain36/1 -> Gain29/1
  Gain24/1 -> Gain32/1
  Demux2/8 -> Subsystem8/1(In1)
  Subsystem1/1(F_gated) -> Gain/1
  Gain37/1 -> Gain30/1
  Subsystem4/1(F_gated) -> Gain38/1
  Gain/1 -> Gain28/1
  Subsystem8/1(F_gated) -> Gain27/1
  Gain25/1 -> Gain33/1
  Demux2/2 -> Subsystem2/1(In1)
  Subsystem5/1(F_gated) -> Gain24/1
  Demux2/1 -> Subsystem1/1(In1)
  Command Switch1/2(tau_cmd) -> RCS_Force_Torque_Allocation1/2(tau_cmd)
  From79/1 -> Gain20/1
  Constant40/1 -> Degrees to Radians4/1
  Gain23/1 -> SS Attitude Control wrt ECI/4(Kp_rw)
  Quaternion Multiplication1/1 -> SS Attitude Control wrt ECI/1(q_err), Quaternions to Rotation Angles2/1
  SS Attitude Control wrt ECI/1(RW_cmd) -> Gain10/1
  Manual Switch6/1 -> RCS_Position&Attitude_Controller1/12(Kp_pos)
  Constant52/1 -> RCS_Force_Torque_Allocation1/4(RCS_F_vec)
  Constant14/1 -> Gain22/1
  Constant32/1 -> Manual Switch5/2
  Manual Switch1/1 -> RCS_Position&Attitude_Controller1/3(r_ref)
  From77/1 -> Manual Switch5/1
  Radians to Degrees5/1 -> attitude error/1
  From6/1 -> Quaternion Multiplication1/1
  Gain7/1 -> Manual Switch7/2
  Gain39/1 -> SS Attitude Control wrt ECI/5(Kd_rw)
  From4/1 -> Product1/1
  From75/1 -> Quaternion Multiplication4/2
  Command Switch1/1(F_cmd) -> Gain21/1
  Gain22/1 -> RCS_Position&Attitude_Controller1/14(Kp_att)
  Constant10/1 -> Gain7/1
  Manual Switch7/1 -> RCS_Position&Attitude_Controller1/13(Kd_pos)
  Gain4/1 -> Manual Switch6/1
  Quaternion Multiplication4/1 -> RCS_Position&Attitude_Controller1/7(q_err)
  Degrees to Radians5/1 -> Add4/1
  Constant15/1 -> RCS_Position&Attitude_Controller1/10(m_sc)
  Gain12/1 -> Command Switch1/2(tau_PD_cmd)
  Constant41/1 -> Degrees to Radians5/1
  Add10/1 -> Radians to Degrees6/1, SS Attitude Control wrt ECI/2(w_err)
  Constant30/1 -> Gain18/1
  Quaternions to Rotation Angles2/1 -> Radians to Degrees5/1
  From5/1 -> Add10/1
  Constant31/1 -> Manual Switch1/2
  Gain21/1 -> RCS_Force_Torque_Allocation1/1(F_cmd)
  Constant34/1 -> RCS_Force_Torque_Allocation1/5(Tmax)
  Gain11/1 -> Manual Switch6/2
  Rotation Angles to Quaternions4/1 -> Quaternion Multiplication4/1
  From12/1 -> Add4/2, RCS_Position&Attitude_Controller1/9(wb)
  Constant13/1 -> Gain3/1
  Constant9/1 -> Gain11/1
  From40/1 -> Add10/2
  Constant11/1 -> Gain23/1
  RCS_Force_Torque_Allocation1/1(duty) -> Goto33/1
  Add4/1 -> RCS_Position&Attitude_Controller1/8("w_err ")
  From9/1 -> RCS_Position&Attitude_Controller1/1(r_rel)
  From76/1 -> Command Switch1/3(F_QP_cmd)
  From70/1 -> RCS_Position&Attitude_Controller1/2(v_rel)
  Constant35/1 -> RCS_Force_Torque_Allocation1/6(wF)
  From68/1 -> Command Switch1/5(flag)
  From71/1 -> RCS_Position&Attitude_Controller1/6("q ")
  Degrees to Radians4/1 -> Rotation Angles to Quaternions4/1
  Gain3/1 -> SS Attitude Control wrt ECI/6(Ki_rw)
  RCS_Position&Attitude_Controller1/2(tau_cmd_B) -> Gain12/1
  Constant33/1 -> RCS_Position&Attitude_Controller1/11(Ib)
  From74/1 -> Manual Switch1/1
  From8/1 -> attitude error/3
  Radians to Degrees6/1 -> attitude error/2
  Manual Switch5/1 -> RCS_Position&Attitude_Controller1/4(v_ref)
  RCS_Position&Attitude_Controller1/1(F_cmd_B) -> Gain8/1
  Gain8/1 -> Command Switch1/1(F_PD_cmd)
  From73/1 -> Command Switch1/4(tau_QP_cmd)
  Constant36/1 -> SS Attitude Control wrt ECI/3(As)
  From78/1 -> Gain4/1
  Constant23/1 -> RCS_Position&Attitude_Controller1/5(a_ref)
  Product1/1 -> Goto32/1
  Gain18/1 -> RCS_Position&Attitude_Controller1/15(Kd_att)
  Gain20/1 -> Manual Switch7/1
  From7/1 -> Quaternion Inverse1/1
  Constant49/1 -> RCS_Force_Torque_Allocation1/3(RCS_pos)
  Constant39/1 -> RCS_Force_Torque_Allocation1/7(wT)
  Gain10/1 -> Product1/2
  Constant12/1 -> Gain39/1
  Quaternion Inverse1/1 -> Quaternion Multiplication1/2

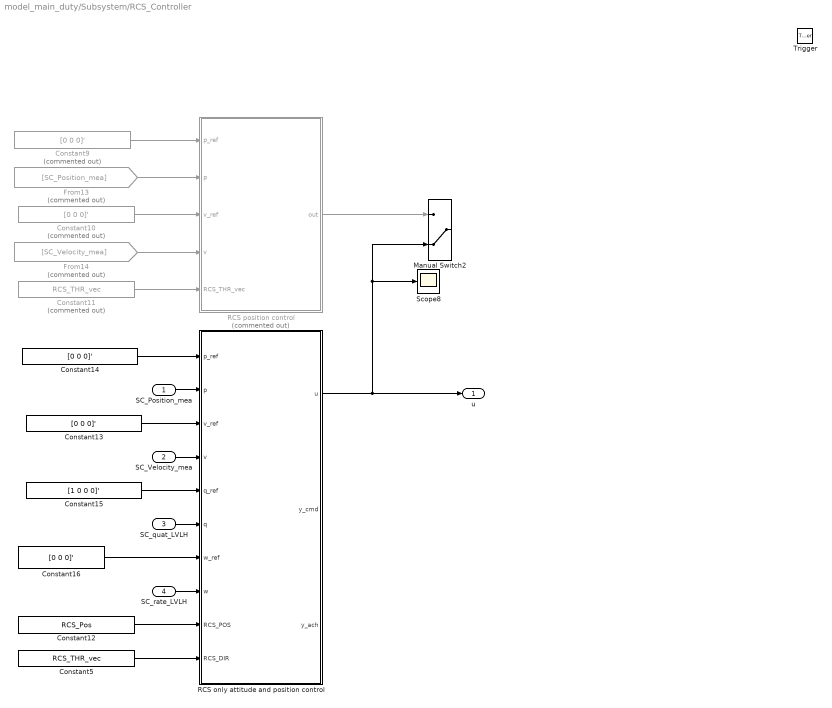
== system model_main_duty/Subsystem/RCS_Controller ==
  SC_Position_mea : Inport
  SC_Velocity_mea : Inport  Port=2
  SC_quat_LVLH : Inport  Port=3
  SC_rate_LVLH : Inport  Port=4
  Trigger : TriggerPort  TriggerType=either  VariantControl=(inherit)  PortDimensions=1
  Constant10 : Constant  Commented=on  Value=[0 0 0]'
  Constant11 : Constant  Commented=on  Value=RCS_THR_vec
  Constant12 : Constant  Value=RCS_Pos
  Constant13 : Constant  Value=[0 0 0]'
  Constant14 : Constant  Value=[0 0 0]'
  Constant15 : Constant  Value=[1 0 0 0]'
  Constant16 : Constant  Value=[0 0 0]'
  Constant5 : Constant  Value=RCS_THR_vec
  Constant9 : Constant  Commented=on  Value=[0 0 0]'
  From13 : From  Commented=on  GotoTag=SC_Position_mea  TagVisibility=global
  From14 : From  Commented=on  GotoTag=SC_Velocity_mea  TagVisibility=global
  Manual Switch2 : ManualSwitch  CurrentSetting=0
  RCS only attitude and position control : MATLAB Function  TreatAsAtomicUnit=on
  RCS position control : MATLAB Function  Commented=on  TreatAsAtomicUnit=on
  Scope8 : Scope
  u : Outport
  wires:
  Constant5/1 -> RCS only attitude and position control/10(RCS_DIR)
  SC_quat_LVLH/1 -> RCS only attitude and position control/6(q)
  Constant12/1 -> RCS only attitude and position control/9(RCS_POS)
  SC_rate_LVLH/1 -> RCS only attitude and position control/8(w)
  SC_Velocity_mea/1 -> RCS only attitude and position control/4(v)
  From13/1 -> RCS position control/2(p)
  RCS only attitude and position control/1(u) -> Manual Switch2/2, Scope8/1, u/1
  Constant13/1 -> RCS only attitude and position control/3(v_ref)
  Constant15/1 -> RCS only attitude and position control/5(q_ref)
  RCS position control/1(out) -> Manual Switch2/1
  Constant16/1 -> RCS only attitude and position control/7(w_ref)
  Constant10/1 -> RCS position control/3(v_ref)
  Constant9/1 -> RCS position control/1(p_ref)
  Constant11/1 -> RCS position control/5(RCS_THR_vec)
  SC_Position_mea/1 -> RCS only attitude and position control/2(p)
  Constant14/1 -> RCS only attitude and position control/1(p_ref)
  From14/1 -> RCS position control/4(v)

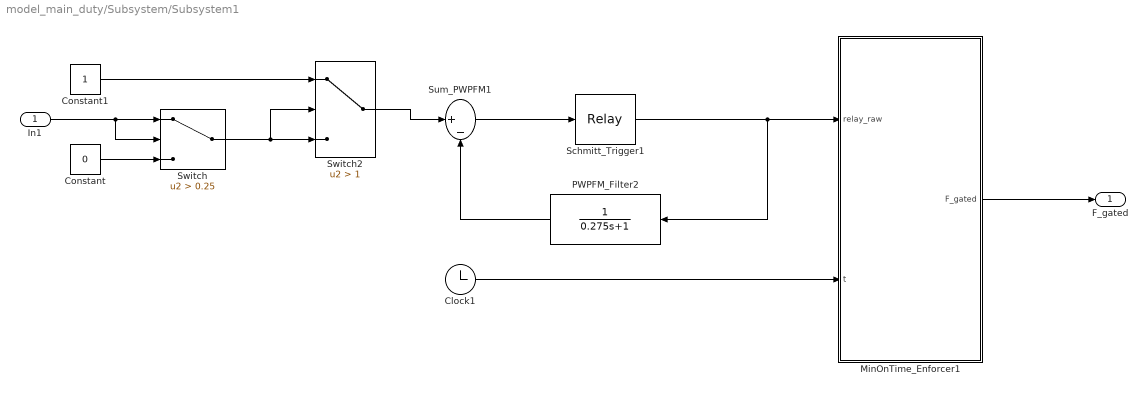
== system model_main_duty/Subsystem/Subsystem1 ==
  In1 : Inport
  Clock1 : Clock
  Constant : Constant  Value=0
  Constant1 : Constant
  MinOnTime_Enforcer1 : MATLAB Function  TreatAsAtomicUnit=on
  PWPFM_Filter2 : TransferFcn  Numerator=1  Denominator=[0.275 1]
  Schmitt_Trigger1 : Relay  OnSwitchValue=0.127  OffSwitchValue=-0.127
  Sum_PWPFM1 : Sum  Inputs=|+-
  Switch : Switch  Criteria=u2 > Threshold  Threshold=0.25  SaturateOnIntegerOverflow=off  InputSameDT=off
  Switch2 : Switch  Criteria=u2 > Threshold  Threshold=1  SaturateOnIntegerOverflow=off  InputSameDT=off
  F_gated : Outport
  wires:
  Schmitt_Trigger1/1 -> MinOnTime_Enforcer1/1(relay_raw), PWPFM_Filter2/1
  PWPFM_Filter2/1 -> Sum_PWPFM1/2
  Sum_PWPFM1/1 -> Schmitt_Trigger1/1
  MinOnTime_Enforcer1/1(F_gated) -> F_gated/1
  Clock1/1 -> MinOnTime_Enforcer1/2(t)
  Switch2/1 -> Sum_PWPFM1/1
  Constant1/1 -> Switch2/1
  Switch/1 -> Switch2/3, Switch2/2
  Constant/1 -> Switch/3
  In1/1 -> Switch/1, Switch/2

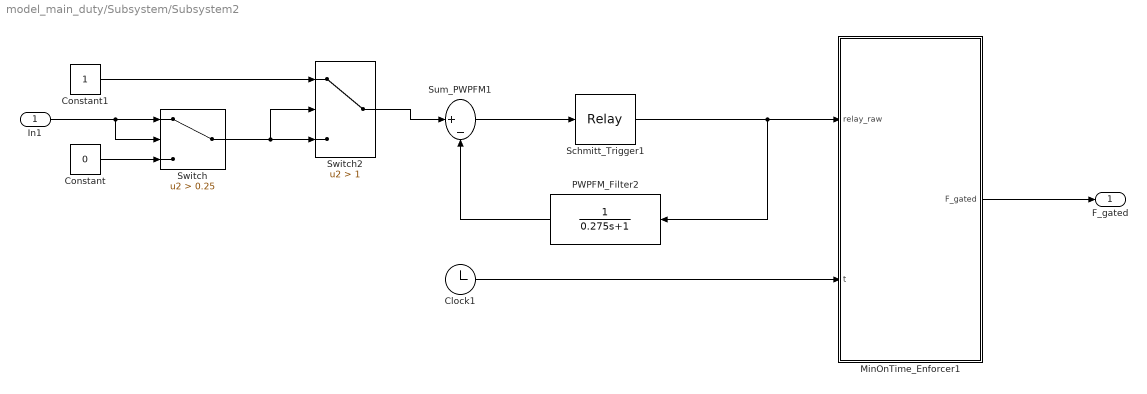
== system model_main_duty/Subsystem/Subsystem2 ==
  In1 : Inport
  Clock1 : Clock
  Constant : Constant  Value=0
  Constant1 : Constant
  MinOnTime_Enforcer1 : MATLAB Function  TreatAsAtomicUnit=on
  PWPFM_Filter2 : TransferFcn  Numerator=1  Denominator=[0.275 1]
  Schmitt_Trigger1 : Relay  OnSwitchValue=0.127  OffSwitchValue=-0.127
  Sum_PWPFM1 : Sum  Inputs=|+-
  Switch : Switch  Criteria=u2 > Threshold  Threshold=0.25  SaturateOnIntegerOverflow=off  InputSameDT=off
  Switch2 : Switch  Criteria=u2 > Threshold  Threshold=1  SaturateOnIntegerOverflow=off  InputSameDT=off
  F_gated : Outport
  wires:
  Schmitt_Trigger1/1 -> MinOnTime_Enforcer1/1(relay_raw), PWPFM_Filter2/1
  PWPFM_Filter2/1 -> Sum_PWPFM1/2
  Sum_PWPFM1/1 -> Schmitt_Trigger1/1
  MinOnTime_Enforcer1/1(F_gated) -> F_gated/1
  Clock1/1 -> MinOnTime_Enforcer1/2(t)
  Switch2/1 -> Sum_PWPFM1/1
  Constant1/1 -> Switch2/1
  Switch/1 -> Switch2/3, Switch2/2
  Constant/1 -> Switch/3
  In1/1 -> Switch/1, Switch/2

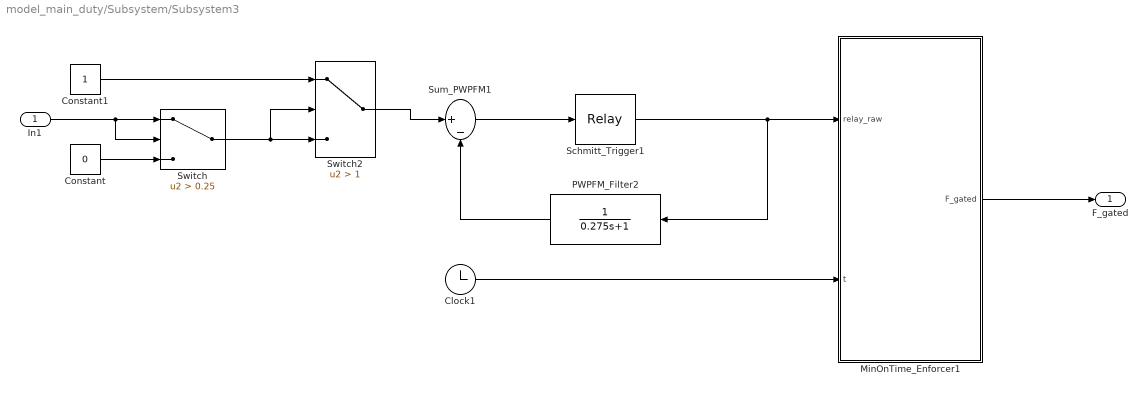
== system model_main_duty/Subsystem/Subsystem3 ==
  In1 : Inport
  Clock1 : Clock
  Constant : Constant  Value=0
  Constant1 : Constant
  MinOnTime_Enforcer1 : MATLAB Function  TreatAsAtomicUnit=on
  PWPFM_Filter2 : TransferFcn  Numerator=1  Denominator=[0.275 1]
  Schmitt_Trigger1 : Relay  OnSwitchValue=0.127  OffSwitchValue=-0.127
  Sum_PWPFM1 : Sum  Inputs=|+-
  Switch : Switch  Criteria=u2 > Threshold  Threshold=0.25  SaturateOnIntegerOverflow=off  InputSameDT=off
  Switch2 : Switch  Criteria=u2 > Threshold  Threshold=1  SaturateOnIntegerOverflow=off  InputSameDT=off
  F_gated : Outport
  wires:
  Schmitt_Trigger1/1 -> MinOnTime_Enforcer1/1(relay_raw), PWPFM_Filter2/1
  PWPFM_Filter2/1 -> Sum_PWPFM1/2
  Sum_PWPFM1/1 -> Schmitt_Trigger1/1
  MinOnTime_Enforcer1/1(F_gated) -> F_gated/1
  Clock1/1 -> MinOnTime_Enforcer1/2(t)
  Switch2/1 -> Sum_PWPFM1/1
  Constant1/1 -> Switch2/1
  Switch/1 -> Switch2/3, Switch2/2
  Constant/1 -> Switch/3
  In1/1 -> Switch/1, Switch/2

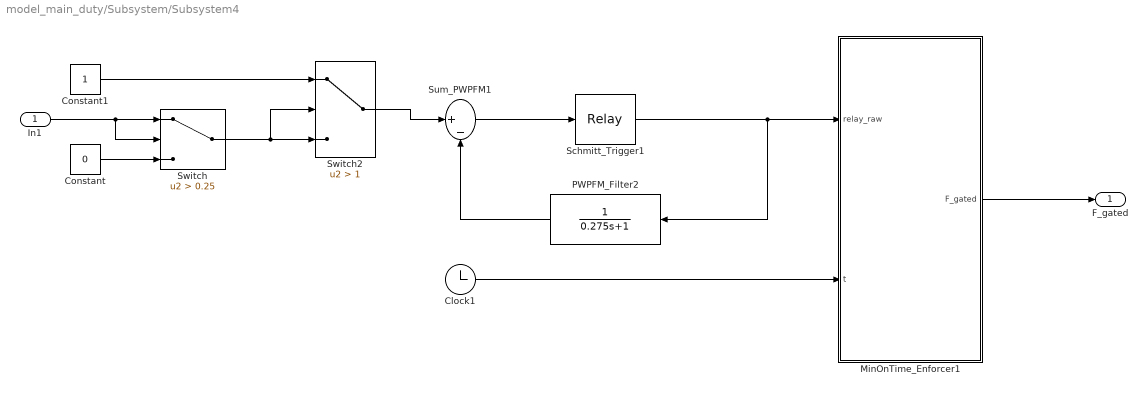
== system model_main_duty/Subsystem/Subsystem4 ==
  In1 : Inport
  Clock1 : Clock
  Constant : Constant  Value=0
  Constant1 : Constant
  MinOnTime_Enforcer1 : MATLAB Function  TreatAsAtomicUnit=on
  PWPFM_Filter2 : TransferFcn  Numerator=1  Denominator=[0.275 1]
  Schmitt_Trigger1 : Relay  OnSwitchValue=0.127  OffSwitchValue=-0.127
  Sum_PWPFM1 : Sum  Inputs=|+-
  Switch : Switch  Criteria=u2 > Threshold  Threshold=0.25  SaturateOnIntegerOverflow=off  InputSameDT=off
  Switch2 : Switch  Criteria=u2 > Threshold  Threshold=1  SaturateOnIntegerOverflow=off  InputSameDT=off
  F_gated : Outport
  wires:
  Schmitt_Trigger1/1 -> MinOnTime_Enforcer1/1(relay_raw), PWPFM_Filter2/1
  PWPFM_Filter2/1 -> Sum_PWPFM1/2
  Sum_PWPFM1/1 -> Schmitt_Trigger1/1
  MinOnTime_Enforcer1/1(F_gated) -> F_gated/1
  Clock1/1 -> MinOnTime_Enforcer1/2(t)
  Switch2/1 -> Sum_PWPFM1/1
  Constant1/1 -> Switch2/1
  Switch/1 -> Switch2/3, Switch2/2
  Constant/1 -> Switch/3
  In1/1 -> Switch/1, Switch/2

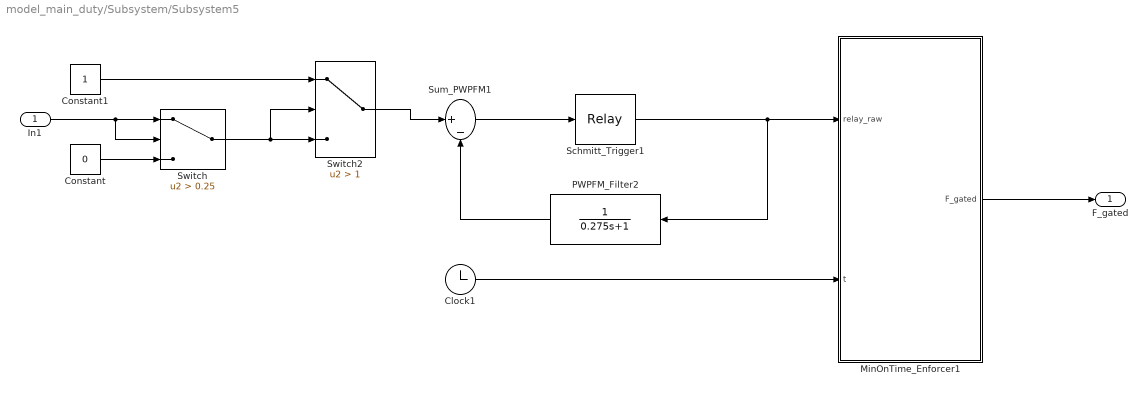
== system model_main_duty/Subsystem/Subsystem5 ==
  In1 : Inport
  Clock1 : Clock
  Constant : Constant  Value=0
  Constant1 : Constant
  MinOnTime_Enforcer1 : MATLAB Function  TreatAsAtomicUnit=on
  PWPFM_Filter2 : TransferFcn  Numerator=1  Denominator=[0.275 1]
  Schmitt_Trigger1 : Relay  OnSwitchValue=0.127  OffSwitchValue=-0.127
  Sum_PWPFM1 : Sum  Inputs=|+-
  Switch : Switch  Criteria=u2 > Threshold  Threshold=0.25  SaturateOnIntegerOverflow=off  InputSameDT=off
  Switch2 : Switch  Criteria=u2 > Threshold  Threshold=1  SaturateOnIntegerOverflow=off  InputSameDT=off
  F_gated : Outport
  wires:
  Schmitt_Trigger1/1 -> MinOnTime_Enforcer1/1(relay_raw), PWPFM_Filter2/1
  PWPFM_Filter2/1 -> Sum_PWPFM1/2
  Sum_PWPFM1/1 -> Schmitt_Trigger1/1
  MinOnTime_Enforcer1/1(F_gated) -> F_gated/1
  Clock1/1 -> MinOnTime_Enforcer1/2(t)
  Switch2/1 -> Sum_PWPFM1/1
  Constant1/1 -> Switch2/1
  Switch/1 -> Switch2/3, Switch2/2
  Constant/1 -> Switch/3
  In1/1 -> Switch/1, Switch/2
